simulink model "sampleModel1555"  (R2023a)
settings: Solver=VariableStepAuto  StartTime=0.0  StopTime=10.0  RelTol=1e-3
libraries: hdlsllib x3, simulink x1
settings Model: Creator=user1  LastModifiedBy=user1

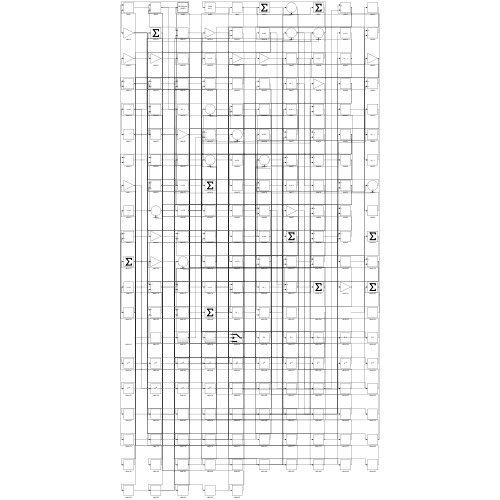
[thumbnail: Simulink's stored preview of the top-level diagram]
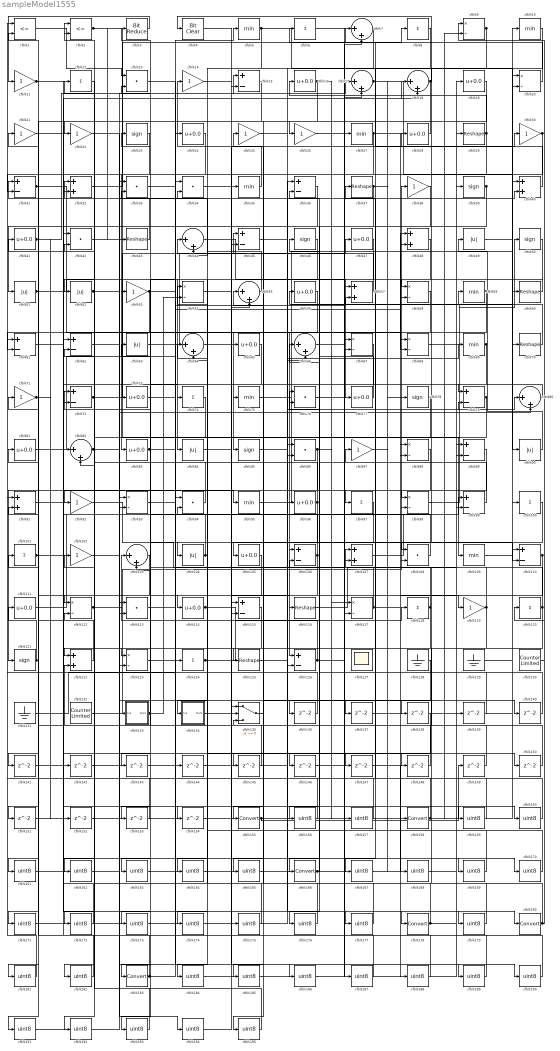
== system sampleModel1555 ==
  cfblk1 : RelationalOperator  Operator=<=  OutDataTypeStr=boolean  InputSameDT=off
  cfblk{5,10,27,35,59,69,75,95,109} (9 alike) : MinMax
  cfblk{6,8,12,74,97,100..101,118,120,124} (10 alike) : Sum  Inputs=+
  cfblk{11,14,21..22,25..26,30,38,53,71,87,92,102,119} (14 alike) : Gain
  cfblk{7,17..18,44,55,64,66,80,82,103} (10 alike) : Sum  Inputs=|++
  cfblk{49,51..52,63,84,90,104} (7 alike) : Abs  SaturateOnIntegerOverflow=off
  cfblk{16,19,24,28,41,47,56,65,73,77,81,83,96,105,111,114} (16 alike) : Bias  Bias=0.0  SaturateOnIntegerOverflow=off
  cfblk{15,31,36,45,61..62,72,79,89,99,106,110,115,126} (14 alike) : Sum  Inputs=+-
  cfblk{32,40,48,57,91,107,122} (7 alike) : Sum
  cfblk{13,33..34,42,76,86,94,108,113} (9 alike) : DotProduct  OutDataTypeStr=Inherit: Inherit via internal rule
  cfblk{9,20,54,58,67..68,88,93,98,112,117,123} (12 alike) : Product  Inputs=*/  RndMeth=Zero  SaturateOnIntegerOverflow=on
  cfblk{29,37,43,60,70,116,125} (7 alike) : Reshape
  cfblk{23,39,46,50,78,85,121} (7 alike) : Signum
  cfblk127 : Scope
      settings: Floating=on
  cfblk128 : Ground
  cfblk129 : Ground
  cfblk130 : hdlsllib/Sources/Counter Limited  uplimit=7  tsamp=-1
  cfblk131 : Ground
  cfblk132 : hdlsllib/Sources/Counter Limited  uplimit=7  tsamp=-1
  cfblk133 : Subsystem
      settings: LibrarySourceBlock=|
      | hdlsllib/Ports &
      | Subsystems/Subsystem
  cfblk134 : Subsystem
      settings: LibrarySourceBlock=|
      | hdlsllib/Ports &
      | Subsystems/Subsystem
  cfblk135 : Switch  SaturateOnIntegerOverflow=off  InputSameDT=off
  cfblk{136..154} (19 alike) : Delay  SampleTime=1
  cfblk{155,158,166,178,180,183} (6 alike) : DataTypeConversion  SaturateOnIntegerOverflow=off  RndMeth=Floor
  cfblk{156..157,159..165,167..177,179,181..182,184..195} (35 alike) : DataTypeConversion  OutDataTypeStr=uint8  SaturateOnIntegerOverflow=off  RndMeth=Floor
  cfblk2 : RelationalOperator  Operator=<=  OutDataTypeStr=boolean  InputSameDT=off
  cfblk3 : hdlsllib/Logic and Bit Operations/Bit Reduce  mode=AND
  cfblk4 : simulink/Logic and Bit Operations/Bit Clear  iBit=0
      settings: LibrarySourceBlock=|
      | hdlsllib/Logic and Bit
      | Operations/Bit Clear
  wires:
  cfblk37/1 -> cfblk168/1, cfblk176/1
  cfblk30/1 -> cfblk104/1, cfblk31/2
  cfblk92/1 -> cfblk107/1
  cfblk67/1 -> cfblk183/1
  cfblk63/1 -> cfblk45/1
  cfblk24/1 -> cfblk83/1
  cfblk72/1 -> cfblk47/1, cfblk80/2
  cfblk29/1 -> cfblk16/1, cfblk161/1
  cfblk41/1 -> cfblk15/1, cfblk142/1
  cfblk95/1 -> cfblk59/1
  cfblk130/1 -> cfblk9/1
  cfblk35/1 -> cfblk14/1
  cfblk86/1 -> cfblk121/1, cfblk157/1
  cfblk97/1 -> cfblk105/1
  cfblk131/1 -> cfblk94/1
  cfblk88/1 -> cfblk92/1
  cfblk58/1 -> cfblk85/1
  cfblk11/1 -> cfblk74/1, cfblk147/1, cfblk177/1
  cfblk98/1 -> cfblk50/1
  cfblk90/1 -> cfblk49/1
  cfblk2/1 -> cfblk109/1, cfblk43/1
  cfblk84/1 -> cfblk107/2
  cfblk36/1 -> cfblk155/1
  cfblk47/1 -> cfblk84/1
  cfblk3/1 -> cfblk11/1
  cfblk126/1 -> cfblk103/1, cfblk7/2
  cfblk135/1 -> cfblk55/1
  cfblk59/1 -> cfblk126/1, cfblk164/1, cfblk182/1
  cfblk32/1 -> cfblk8/1
  cfblk51/1 -> cfblk53/1, cfblk18/2
  cfblk83/1 -> cfblk5/1, cfblk57/2, cfblk58/2
  cfblk18/1 -> cfblk4/1, cfblk26/1
  cfblk53/1 -> cfblk61/2, cfblk136/1
  cfblk132/1 -> cfblk27/1
  cfblk112/1 -> cfblk98/2, cfblk148/1
  cfblk49/1 -> cfblk60/1
  cfblk108/1 -> cfblk54/1
  cfblk50/1 -> cfblk134/1(In1)
  cfblk65/1 -> cfblk75/1
  cfblk129/1 -> cfblk20/2
  cfblk5/1 -> cfblk90/1, cfblk15/2
  cfblk28/1 -> cfblk22/1
  cfblk77/1 -> cfblk46/1
  cfblk111/1 -> cfblk38/1
  cfblk80/1 -> cfblk79/1
  cfblk17/1 -> cfblk70/1, cfblk78/1
  cfblk68/1 -> cfblk10/1
  cfblk71/1 -> cfblk151/1, cfblk152/1
  cfblk57/1 -> cfblk44/1
  cfblk42/1 -> cfblk124/1
  cfblk8/1 -> cfblk97/1
  cfblk54/1 -> cfblk116/1
  cfblk94/1 -> cfblk2/1
  cfblk60/1 -> cfblk58/1
  cfblk31/1 -> cfblk96/1, cfblk73/1
  cfblk114/1 -> cfblk118/1, cfblk30/1
  cfblk104/1 -> cfblk64/1, cfblk3/1
  cfblk46/1 -> cfblk123/1
  cfblk134/1(Out1) -> cfblk65/1
  cfblk74/1 -> cfblk112/1
  cfblk110/1 -> cfblk122/1, cfblk184/1
  cfblk75/1 -> cfblk40/1
  cfblk100/1 -> cfblk106/1
  cfblk44/1 -> cfblk77/1
  cfblk55/1 -> cfblk31/1
  cfblk85/1 -> cfblk69/1
  cfblk105/1 -> cfblk114/1
  cfblk64/1 -> cfblk35/1
  cfblk117/1 -> cfblk119/1, cfblk64/2
  cfblk45/1 -> cfblk110/2
  cfblk124/1 -> cfblk88/2, cfblk28/1
  cfblk91/1 -> cfblk180/1
  cfblk52/1 -> cfblk17/1, cfblk150/1
  cfblk99/1 -> cfblk76/1
  cfblk118/1 -> cfblk125/1, cfblk72/2
  cfblk27/1 -> cfblk68/1, cfblk32/2
  cfblk101/1 -> cfblk99/1, cfblk154/1
  cfblk43/1 -> cfblk21/1
  cfblk89/1 -> cfblk166/1
  cfblk121/1 -> cfblk111/1, cfblk191/1
  cfblk40/1 -> cfblk7/1
  cfblk76/1 -> cfblk79/2
  cfblk10/1 -> cfblk86/2
  cfblk9/1 -> cfblk44/2, cfblk108/1
  cfblk79/1 -> cfblk123/2, cfblk82/2
  cfblk116/1 -> cfblk19/1
  cfblk109/1 -> cfblk100/1
  cfblk38/1 -> cfblk51/1
  cfblk87/1 -> cfblk158/1
  cfblk70/1 -> cfblk56/1
  cfblk25/1 -> cfblk178/1
  cfblk106/1 -> cfblk63/1, cfblk162/1
  cfblk133/1(Out1) -> cfblk33/2, cfblk23/1, cfblk54/2
  cfblk69/1 -> cfblk153/1, cfblk167/1
  cfblk39/1 -> cfblk57/1, cfblk165/1
  cfblk120/1 -> cfblk32/1, cfblk156/1
  cfblk82/1 -> cfblk40/2, cfblk145/1
  cfblk16/1 -> cfblk52/1, cfblk117/1, cfblk185/1
  cfblk96/1 -> cfblk41/1, cfblk143/1
  cfblk13/1 -> cfblk68/2
  cfblk81/1 -> cfblk18/1
  cfblk125/1 -> cfblk80/1
  cfblk21/1 -> cfblk82/1
  cfblk19/1 -> cfblk98/1
  cfblk61/1 -> cfblk95/1
  cfblk1/1 -> cfblk13/1
  cfblk107/1 -> cfblk39/1
  cfblk7/1 -> cfblk135/2
  cfblk119/1 -> cfblk135/3, cfblk72/1
  cfblk20/1 -> cfblk6/1
  cfblk122/1 -> cfblk81/1
  cfblk136/1 -> cfblk1/1
  cfblk33/1 -> cfblk137/1
  cfblk137/1 -> cfblk110/1
  cfblk123/1 -> cfblk138/1
  cfblk139/1 -> cfblk88/1
  cfblk22/1 -> cfblk140/1
  cfblk140/1 -> cfblk106/2
  cfblk15/1 -> cfblk141/1
  cfblk142/1 -> cfblk45/2
  cfblk143/1 -> cfblk55/2
  cfblk73/1 -> cfblk144/1
  cfblk144/1 -> cfblk86/1
  cfblk145/1 -> cfblk103/2
  cfblk14/1 -> cfblk146/1
  cfblk146/1 -> cfblk17/2
  cfblk148/1 -> cfblk1/2
  cfblk149/1 -> cfblk13/2
  cfblk150/1 -> cfblk122/2
  cfblk151/1 -> cfblk126/2
  cfblk152/1 -> cfblk2/2
  cfblk153/1 -> cfblk61/1
  cfblk155/1 -> cfblk149/1, cfblk20/1
  cfblk156/1 -> cfblk36/1
  cfblk157/1 -> cfblk36/2
  cfblk158/1 -> cfblk101/1, cfblk9/2
  cfblk154/1 -> cfblk159/1
  cfblk159/1 -> cfblk87/1
  cfblk113/1 -> cfblk160/1
  cfblk160/1 -> cfblk37/1
  cfblk161/1 -> cfblk113/1
  cfblk162/1 -> cfblk113/2
  cfblk48/1 -> cfblk163/1
  cfblk163/1 -> cfblk139/1
  cfblk164/1 -> cfblk48/1
  cfblk165/1 -> cfblk48/2
  cfblk166/1 -> cfblk117/2, cfblk76/2
  cfblk167/1 -> cfblk89/1
  cfblk168/1 -> cfblk89/2
  cfblk66/1 -> cfblk169/1
  cfblk169/1 -> cfblk94/2
  cfblk141/1 -> cfblk170/1
  cfblk170/1 -> cfblk66/1
  cfblk103/1 -> cfblk171/1
  cfblk171/1 -> cfblk66/2
  cfblk115/1 -> cfblk172/1
  cfblk172/1 -> cfblk42/1
  cfblk56/1 -> cfblk173/1
  cfblk173/1 -> cfblk115/1
  cfblk138/1 -> cfblk174/1
  cfblk174/1 -> cfblk115/2
  cfblk34/1 -> cfblk175/1
  cfblk175/1 -> cfblk42/2
  cfblk176/1 -> cfblk34/1
  cfblk177/1 -> cfblk34/2
  cfblk178/1 -> cfblk99/2, cfblk112/2
  cfblk6/1 -> cfblk179/1
  cfblk179/1 -> cfblk25/1
  cfblk180/1 -> cfblk108/2, cfblk120/1
  cfblk23/1 -> cfblk181/1
  cfblk181/1 -> cfblk91/1
  cfblk182/1 -> cfblk91/2
  cfblk183/1 -> cfblk24/1, cfblk71/1
  cfblk184/1 -> cfblk67/1
  cfblk185/1 -> cfblk67/2
  cfblk62/1 -> cfblk186/1
  cfblk186/1 -> cfblk29/1
  cfblk26/1 -> cfblk187/1
  cfblk187/1 -> cfblk62/1
  cfblk147/1 -> cfblk188/1
  cfblk188/1 -> cfblk62/2
  cfblk93/1 -> cfblk189/1
  cfblk189/1 -> cfblk33/1
  cfblk4/1 -> cfblk190/1
  cfblk190/1 -> cfblk93/1
  cfblk191/1 -> cfblk93/2
  cfblk12/1 -> cfblk192/1
  cfblk192/1 -> cfblk133/1(In1)
  cfblk78/1 -> cfblk193/1
  cfblk193/1 -> cfblk12/1
  cfblk102/1 -> cfblk194/1
  cfblk194/1 -> cfblk135/1
  cfblk128/1 -> cfblk195/1
  cfblk195/1 -> cfblk102/1

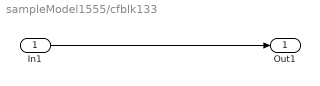
== system sampleModel1555/cfblk133 ==
  In1 : Inport
  Out1 : Outport
  wires:
  In1/1 -> Out1/1

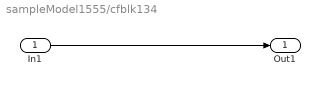
== system sampleModel1555/cfblk134 ==
  In1 : Inport
  Out1 : Outport
  wires:
  In1/1 -> Out1/1
